simulink model "ThdRwRtStCalib"  (R2024b)
settings: Solver=FixedStepDiscrete  StartTime=0.0  StopTime=10.0  FixedStep=0.01  RelTol=1e-3
model workspace (MAT data in the model file):
  KeSMSwAcsMd7ThdRwRtStBkReclnUpwdDnwdPosMax_Val = Simulink.Parameter
  KeSMSwAcsMd7ThdRwRtStBkReclnUpwdDnwdPosMax_Val.Value = 0
  KeSMSwAcsMd7ThdRwRtStBkReclnUpwdDnwdPosMax_Val.Complexity = 'real'
  KeSMSwAcsMd7ThdRwRtStBkReclnUpwdDnwdPosMax_Val.Dimensions = [1 1]
  KeSMSwAcsMd7ThdRwRtStBkReclnUpwdDnwdPosMax_Val.DataType = 'uint16'
  KeSMSwAcsMd7ThdRwRtStBkReclnUpwdDnwdPosMin_Val = Simulink.Parameter
  KeSMSwAcsMd7ThdRwRtStBkReclnUpwdDnwdPosMin_Val.Value = 0
  KeSMSwAcsMd7ThdRwRtStBkReclnUpwdDnwdPosMin_Val.Complexity = 'real'
  KeSMSwAcsMd7ThdRwRtStBkReclnUpwdDnwdPosMin_Val.Dimensions = [1 1]
  KeSMSwAcsMd7ThdRwRtStBkReclnUpwdDnwdPosMin_Val.DataType = 'uint16'
  KeSMSwAcsMd7ThdRwRtStBkReclnUpwdDnwdPos_Val = Simulink.Parameter
  KeSMSwAcsMd7ThdRwRtStBkReclnUpwdDnwdPos_Val.Value = 0
  KeSMSwAcsMd7ThdRwRtStBkReclnUpwdDnwdPos_Val.Complexity = 'real'
  KeSMSwAcsMd7ThdRwRtStBkReclnUpwdDnwdPos_Val.Dimensions = [1 1]
  KeSMSwAcsMd7ThdRwRtStBkReclnUpwdDnwdPos_Val.DataType = 'uint16'
  KeSMSwAcsMd7ThdRwRtStCshnFldUpwdDnwdPosMax_Val = Simulink.Parameter
  KeSMSwAcsMd7ThdRwRtStCshnFldUpwdDnwdPosMax_Val.Value = 0
  KeSMSwAcsMd7ThdRwRtStCshnFldUpwdDnwdPosMax_Val.Complexity = 'real'
  KeSMSwAcsMd7ThdRwRtStCshnFldUpwdDnwdPosMax_Val.Dimensions = [1 1]
  KeSMSwAcsMd7ThdRwRtStCshnFldUpwdDnwdPosMax_Val.DataType = 'uint16'
  KeSMSwAcsMd7ThdRwRtStCshnFldUpwdDnwdPosMin_Val = Simulink.Parameter
  KeSMSwAcsMd7ThdRwRtStCshnFldUpwdDnwdPosMin_Val.Value = 0
  KeSMSwAcsMd7ThdRwRtStCshnFldUpwdDnwdPosMin_Val.Complexity = 'real'
  KeSMSwAcsMd7ThdRwRtStCshnFldUpwdDnwdPosMin_Val.Dimensions = [1 1]
  KeSMSwAcsMd7ThdRwRtStCshnFldUpwdDnwdPosMin_Val.DataType = 'uint16'
  KeSMSwAcsMd7ThdRwRtStCshnFldUpwdDnwdPos_Val = Simulink.Parameter
  KeSMSwAcsMd7ThdRwRtStCshnFldUpwdDnwdPos_Val.Value = 0
  KeSMSwAcsMd7ThdRwRtStCshnFldUpwdDnwdPos_Val.Complexity = 'real'
  KeSMSwAcsMd7ThdRwRtStCshnFldUpwdDnwdPos_Val.Dimensions = [1 1]
  KeSMSwAcsMd7ThdRwRtStCshnFldUpwdDnwdPos_Val.DataType = 'uint16'
  KeSMSwAcsMd7ThdRwRtStFrwdBkwdPosMax_Val = Simulink.Parameter
  KeSMSwAcsMd7ThdRwRtStFrwdBkwdPosMax_Val.Value = 0
  KeSMSwAcsMd7ThdRwRtStFrwdBkwdPosMax_Val.Complexity = 'real'
  KeSMSwAcsMd7ThdRwRtStFrwdBkwdPosMax_Val.Dimensions = [1 1]
  KeSMSwAcsMd7ThdRwRtStFrwdBkwdPosMax_Val.DataType = 'uint16'
  KeSMSwAcsMd7ThdRwRtStFrwdBkwdPosMin_Val = Simulink.Parameter
  KeSMSwAcsMd7ThdRwRtStFrwdBkwdPosMin_Val.Value = 0
  KeSMSwAcsMd7ThdRwRtStFrwdBkwdPosMin_Val.Complexity = 'real'
  KeSMSwAcsMd7ThdRwRtStFrwdBkwdPosMin_Val.Dimensions = [1 1]
  KeSMSwAcsMd7ThdRwRtStFrwdBkwdPosMin_Val.DataType = 'uint16'
  KeSMSwAcsMd7ThdRwRtStFrwdBkwdPos_Val = Simulink.Parameter
  KeSMSwAcsMd7ThdRwRtStFrwdBkwdPos_Val.Value = 0
  KeSMSwAcsMd7ThdRwRtStFrwdBkwdPos_Val.Complexity = 'real'
  KeSMSwAcsMd7ThdRwRtStFrwdBkwdPos_Val.Dimensions = [1 1]
  KeSMSwAcsMd7ThdRwRtStFrwdBkwdPos_Val.DataType = 'uint16'
undefined symbols (not defined in the file or in its folder): KeSMSw6sAcsEntryThdRwRtStBkReclnUpwdDnwdPos_Val, KeSMSw6sAcsEntryThdRwRtStBkReclnUpwdDnwdPosMax_Val, KeSMSw6sAcsEntryThdRwRtStBkReclnUpwdDnwdPosMin_Val, KeSMSw6sAcsEntryThdRwRtStCshnFldUpwdDnwdPos_Val, KeSMSw6sAcsEntryThdRwRtStCshnFldUpwdDnwdPosMax_Val, KeSMSw6sAcsEntryThdRwRtStCshnFldUpwdDnwdPosMin_Val, KeSMSw6sAcsEntryThdRwRtStFrwdBkwdPos_Val, KeSMSw6sAcsEntryThdRwRtStFrwdBkwdPosMax_Val, KeSMSw6sAcsEntryThdRwRtStFrwdBkwdPosMin_Val, KeSMSw6SAcsMd56ThdRwRtStBkReclnUpwdDnwdPos_Val, KeSMSw6SAcsMd56ThdRwRtStBkReclnUpwdDnwdPosMax_Val, KeSMSw6SAcsMd56ThdRwRtStBkReclnUpwdDnwdPosMin_Val, KeSMSw6SAcsMd56ThdRwRtStFrwdBkwdPos_Val, KeSMSw6SAcsMd56ThdRwRtStFrwdBkwdPosMax_Val, KeSMSw6SAcsMd56ThdRwRtStFrwdBkwdPosMin_Val, KeSMSw6SAcsMd57ThdRwRtStBkReclnUpwdDnwdPos_Val, KeSMSw6SAcsMd57ThdRwRtStBkReclnUpwdDnwdPosMax_Val, KeSMSw6SAcsMd57ThdRwRtStBkReclnUpwdDnwdPosMin_Val, KeSMSw6SAcsMd57ThdRwRtStFrwdBkwdPos_Val, KeSMSw6SAcsMd57ThdRwRtStFrwdBkwdPosMax_Val, KeSMSw6SAcsMd57ThdRwRtStFrwdBkwdPosMin_Val, KeSMSw6sFamilyMdThdRwRtStFrwdBkwdPos_Val, KeSMSw6sFamilyMdThdRwRtStFrwdBkwdPosMax_Val, KeSMSw6sFamilyMdThdRwRtStFrwdBkwdPosMin_Val, KeSMSw6sFamilyRMdThdRwRtStFrwdBkwdPos_Val, KeSMSw6sFamilyRMdThdRwRtStFrwdBkwdPosMax_Val, KeSMSw6sFamilyRMdThdRwRtStFrwdBkwdPosMin_Val, KeSMSw6sLugThdRwRtStBkReclnUpwdDnwdPos_Val, KeSMSw6sLugThdRwRtStBkReclnUpwdDnwdPosMax_Val, KeSMSw6sLugThdRwRtStBkReclnUpwdDnwdPosMin_Val, KeSMSw6sLugThdRwRtStCshnFldUpwdDnwdPos_Val, KeSMSw6sLugThdRwRtStCshnFldUpwdDnwdPosMax_Val, KeSMSw6sLugThdRwRtStCshnFldUpwdDnwdPosMin_Val, KeSMSw6sLugThdRwRtStFrwdBkwdPos_Val, KeSMSw6sLugThdRwRtStFrwdBkwdPosMax_Val, KeSMSw6sLugThdRwRtStFrwdBkwdPosMin_Val, KeSMSw6sVIPThdRwRtStBkReclnUpwdDnwdPos_Val, KeSMSw6sVIPThdRwRtStBkReclnUpwdDnwdPosMax_Val, KeSMSw6sVIPThdRwRtStBkReclnUpwdDnwdPosMin_Val, KeSMSw6sVIPThdRwRtStFrwdBkwdPos_Val, KeSMSw6sVIPThdRwRtStFrwdBkwdPosMax_Val, KeSMSw6sVIPThdRwRtStFrwdBkwdPosMin_Val, KeSMSwAcsEntryThdRwRtStBkReclnUpwdDnwdPos_Val, KeSMSwAcsEntryThdRwRtStBkReclnUpwdDnwdPosMax_Val, KeSMSwAcsEntryThdRwRtStBkReclnUpwdDnwdPosMin_Val, KeSMSwAcsEntryThdRwRtStCshnFldUpwdDnwdPos_Val, KeSMSwAcsEntryThdRwRtStCshnFldUpwdDnwdPosMax_Val, KeSMSwAcsEntryThdRwRtStCshnFldUpwdDnwdPosMin_Val, KeSMSwAcsEntryThdRwRtStFrwdBkwdPos_Val, KeSMSwAcsEntryThdRwRtStFrwdBkwdPosMax_Val, KeSMSwAcsEntryThdRwRtStFrwdBkwdPosMin_Val, KeSMSwAcsMd53ThdRwRtBkReclnUpwdDnwdPos_Val, KeSMSwAcsMd53ThdRwRtBkReclnUpwdDnwdPosMax_Val, KeSMSwAcsMd53ThdRwRtBkReclnUpwdDnwdPosMin_Val, KeSMSwAcsMd53ThdRwRtFldUpwdDnwdPos_Val, KeSMSwAcsMd53ThdRwRtFldUpwdDnwdPosMax_Val, KeSMSwAcsMd53ThdRwRtFldUpwdDnwdPosMin_Val, KeSMSwAcsMd56ThdRwRtStBkReclnUpwdDnwdPos_Val, KeSMSwAcsMd56ThdRwRtStBkReclnUpwdDnwdPosMax_Val, KeSMSwAcsMd56ThdRwRtStBkReclnUpwdDnwdPosMin_Val ... (+33)
libraries: TrgtPosSelcLib x18
(part 1 of 3)
settings Model: ParameterArgumentNames=KeSMSwAcsMd7ThdRwRtStBkReclnUpwdDnwdPosMax_Val,KeSMSwAcsMd7ThdRwRtStBkReclnUpwdDnwdPosMin_Val,KeSMSwAcsMd7ThdRwRtStBkReclnUpwdDnwdPos_Val,KeSMSwAcsMd7ThdRwRtStCshnFldUpwdDnwdPosMax_Val,KeSMSwAcsMd7ThdRwRtStCshnFldUpwdDnwdPosMin_Val,KeSMSwAcsMd7ThdRwRtStCshnFldUpwdDnwdPos_Val,KeSMSwAcsMd7ThdRwRtStFrwdBkwdPosMax_Val,KeSMSwAcsMd7ThdRwRtStFrwdBkwdPosMin_Val,KeSMSwAcsMd7ThdRwRtStFrwdBkwdPos_Val  Creator=sn2xws  LastModifiedBy=sn55gm
settings Model: ModifiedHistory=|
  | 2024.10.10 V3.5.0 增加Md57 58 增加6sBitMask
  | 2025.3.5 V3.9.0 Bug 998429 LUG模式偶发不会往前移动三排，但是报成功
settings SolverCC: AlgebraicLoopSolver=TrustRegion
settings DataIOCC: SaveFormat=StructureWithTime  ReturnWorkspaceOutputs=off
settings OptimizationCC: DefaultParameterBehavior=Inlined  EnhancedBackFolding=on  PassReuseOutputArgsAs=Individual arguments  ZeroExternalMemoryAtStartup=off  ZeroInternalMemoryAtStartup=off  OptimizeBlockOrder=speed  DifferentSizesBufferReuse=on  OptimizationCustomize=off  EfficientTunableParamExpr=on
settings DebuggingCC: ParameterTunabilityLossMsg=error  UnconnectedInputMsg=warning  UnconnectedOutputMsg=warning  UnconnectedLineMsg=warning  ArithmeticOperatorsInVariantConditions=warning
settings ModelReferenceCC: EnableRefExpFcnMdlSchedulingChecks=on
settings SFSimCC: MATLABDynamicMemAlloc=off  CustomCodeUndefinedFunction=UseInterfaceOnly
settings RTWCC: Description=AUTOSAR  SystemTargetFile=autosar.tlc  GenCodeOnly=on  TemplateMakefile=ert_default_tmf  GenerateReport=on  IncludeHyperlinkInReport=on  LaunchReport=on  DataTypeReplacement=CDataTypesFixedWidth  GenerateTraceInfo=on  GenerateTraceReport=on  GenerateTraceReportSl=on  GenerateTraceReportSf=on  GenerateTraceReportEml=on  GPUComputeCapability=3.5
settings CodeAppCC: ForceParamTrailComments=on  IgnoreCustomStorageClasses=off  OperatorAnnotations=on  SimulinkDataObjDesc=on  SFDataObjDesc=on  InsertBlockDesc=on
settings STFCustomTargetCC: TargetLangStandard=C99 (ISO)  MultiwordLength=256  ParMdlRefBuildCompliant=on  CompOptLevelCompliant=on  IncludeMdlTerminateFcn=off  CombineOutputUpdateFcns=on  SuppressErrorStatus=on  ERTCustomFileBanners=on  SupportNonFinite=off  SupportComplex=off  SupportContinuousTime=off  SupportNonInlinedSFcns=off  RemoveResetFunc=on  MATLABClassNameForMDSCustomization=Simulink.SoftwareTarget.ERTCustomization  AutosarCompliant=on  UseToolchainInfoCompliant=on  LookupTableObjectStructAxisOrder=2,1,3,4,...  LUTObjectStructOrderEvenSpacing=Size,Table,Breakpoints  SystemTargetFile=autosar.tlc
settings ERTTargetCC: TargetLangStandard=C99 (ISO)  ConcurrentExecutionCompliant=off  IncludeMdlTerminateFcn=off  SuppressErrorStatus=on  SupportNonFinite=off  SupportComplex=off  ModelStepFunctionPrototypeControlCompliant=off  CPPClassGenCompliant=off  AutosarCompliant=on  LookupTableObjectStructAxisOrder=2,1,3,4,...  LUTObjectStructOrderEvenSpacing=Size,Table,Breakpoints  ERTCustomFileTemplate=example_file_process.tlc  ERTFilePackagingFormat=Compact  BooleanTrueId=TRUE  BooleanFalseId=FALSE  DynamicArrayContainerType=coder::array

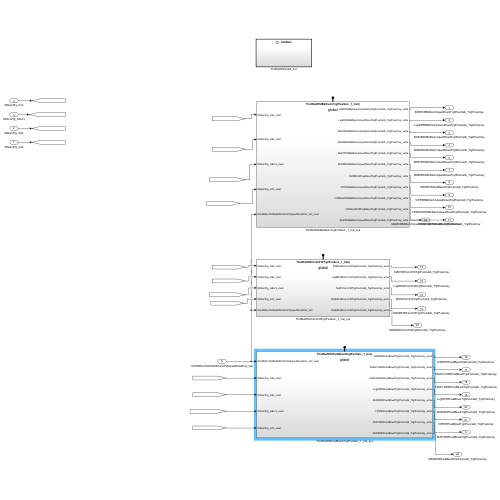
[thumbnail: Simulink's stored preview of the top-level diagram]
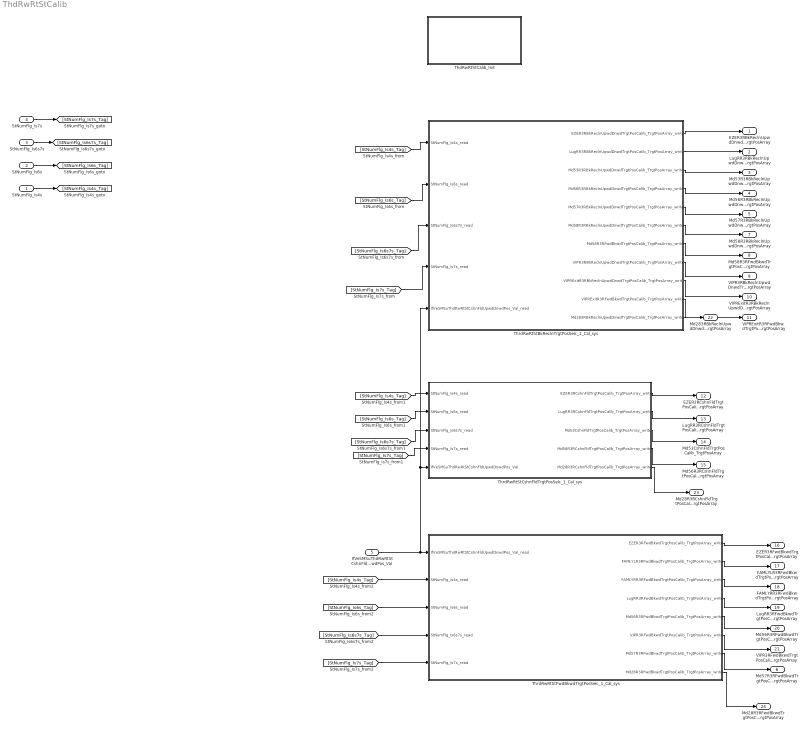
== system ThdRwRtStCalib ==
  StNumFlg_Is4s : Inport  OutDataTypeStr=boolean  PortDimensions=1
  StNumFlg_Is6s : Inport  Port=2  OutDataTypeStr=boolean  PortDimensions=1
  StNumFlg_Is6s7s : Inport  Port=3  OutDataTypeStr=boolean  PortDimensions=1
  StNumFlg_Is7s : Inport  Port=4  OutDataTypeStr=boolean  PortDimensions=1
  IfVeSMSuThdRwRtStCshnFldUpwdDnwdPos_Val : Inport  Port=5  OutDataTypeStr=uint16  PortDimensions=1
  ThdRwRtStCalib_Init : Subsystem
  ThrdRwRtStBkReclnTrgtPosSelc_1_Cal_sys : Subsystem
  ThrdRwRtStCshnFldTrgtPosSelc_1_Cal_sys : Subsystem
  ThrdRwRtStFwdBkwdTrgtPosSelc_1_Cal_sys : Subsystem
  EZER3RBkReclnUpwdDnwdTrgtPosCalib_TrgtPosArray : Outport  Description=|  OutDataTypeStr=uint16  PortDimensions=3  VectorParamsAs1DForOutWhenUnconnected=off
      | 0:Pos
      | 1:Max
      | 2:Min
  LugRR3RBkReclnUpwdDnwdTrgtPosCalib_TrgtPosArray : Outport  Description=|  Port=2  OutDataTypeStr=uint16  PortDimensions=3  VectorParamsAs1DForOutWhenUnconnected=off
      | 0:Pos
      | 1:Max
      | 2:Min
  Md53R3RBkReclnUpwdDnwdTrgtPosCalib_TrgtPosArray : Outport  Description=|  Port=3  OutDataTypeStr=uint16  PortDimensions=3  VectorParamsAs1DForOutWhenUnconnected=off
      | 0:Pos
      | 1:Max
      | 2:Min
  Md56R3RBkReclnUpwdDnwdTrgtPosCalib_TrgtPosArray : Outport  Description=|  Port=4  OutDataTypeStr=uint16  PortDimensions=3  VectorParamsAs1DForOutWhenUnconnected=off
      | 0:Pos
      | 1:Max
      | 2:Min
  Md57R3RBkReclnUpwdDnwdTrgtPosCalib_TrgtPosArray : Outport  Description=|  Port=5  OutDataTypeStr=uint16  PortDimensions=3  VectorParamsAs1DForOutWhenUnconnected=off
      | 0:Pos
      | 1:Max
      | 2:Min
  Md57R3RFwdBkwdTrgtPosCalib_TrgtPosArray : Outport  Description=|  Port=6  OutDataTypeStr=uint16  PortDimensions=3  VectorParamsAs1DForOutWhenUnconnected=off
      | 0:Pos
      | 1:Max
      | 2:Min
  Md58R3RBkReclnUpwdDnwdTrgtPosCalib_TrgtPosArray : Outport  Description=|  Port=7  OutDataTypeStr=uint16  PortDimensions=3  VectorParamsAs1DForOutWhenUnconnected=off
      | 0:Pos
      | 1:Max
      | 2:Min
  Md58R3RFwdBkwdTrgtPosCalib_TrgtPosArray : Outport  Description=|  Port=8  OutDataTypeStr=uint16  PortDimensions=3  VectorParamsAs1DForOutWhenUnconnected=off
      | 0:Pos
      | 1:Max
      | 2:Min
  VIPR3RBkReclnUpwdDnwdTrgtPosCalib_TrgtPosArray : Outport  Description=|  Port=9  OutDataTypeStr=uint16  PortDimensions=3  VectorParamsAs1DForOutWhenUnconnected=off
      | 0:Pos
      | 1:Max
      | 2:Min
  VIPRExitR3RBkReclnUpwdDnwdTrgtPosCalib_TrgtPosArray : Outport  Description=|  Port=10  OutDataTypeStr=uint16  PortDimensions=3  VectorParamsAs1DForOutWhenUnconnected=off
      | 0:Pos
      | 1:Max
      | 2:Min
  VIPRExitR3RFwdBkwdTrgtPosCalib_TrgtPosArray : Outport  Description=|  Port=11  OutDataTypeStr=uint16  PortDimensions=3  VectorParamsAs1DForOutWhenUnconnected=off
      | 0:Pos
      | 1:Max
      | 2:Min
  EZER3RCshnFldTrgtPosCalib_TrgtPosArray : Outport  Description=|  Port=12  OutDataTypeStr=uint16  PortDimensions=3  VectorParamsAs1DForOutWhenUnconnected=off
      | 0:Pos
      | 1:Max
      | 2:Min
  LugRR3RCshnFldTrgtPosCalib_TrgtPosArray : Outport  Description=|  Port=13  OutDataTypeStr=uint16  PortDimensions=3  VectorParamsAs1DForOutWhenUnconnected=off
      | 0:Pos
      | 1:Max
      | 2:Min
  Md53CshnFldTrgtPosCalib_TrgtPosArray : Outport  Description=|  Port=14  OutDataTypeStr=uint16  PortDimensions=3  VectorParamsAs1DForOutWhenUnconnected=off
      | 0:Pos
      | 1:Max
      | 2:Min
  Md56R3RCshnFldTrgtPosCalib_TrgtPosArray : Outport  Description=|  Port=15  OutDataTypeStr=uint16  PortDimensions=3  VectorParamsAs1DForOutWhenUnconnected=off
      | 0:Pos
      | 1:Max
      | 2:Min
  EZER3RFwdBkwdTrgtPosCalib_TrgtPosArray : Outport  Description=|  Port=16  OutDataTypeStr=uint16  PortDimensions=3  VectorParamsAs1DForOutWhenUnconnected=off
      | 0:Pos
      | 1:Max
      | 2:Min
  FAMLYLR3RFwdBkwdTrgtPosCalib_TrgtPosArray : Outport  Description=|  Port=17  OutDataTypeStr=uint16  PortDimensions=3  VectorParamsAs1DForOutWhenUnconnected=off
      | 0:Pos
      | 1:Max
      | 2:Min
  FAMLYRR3RFwdBkwdTrgtPosCalib_TrgtPosArray : Outport  Description=|  Port=18  OutDataTypeStr=uint16  PortDimensions=3  VectorParamsAs1DForOutWhenUnconnected=off
      | 0:Pos
      | 1:Max
      | 2:Min
  LugRR3RFwdBkwdTrgtPosCalib_TrgtPosArray : Outport  Description=|  Port=19  OutDataTypeStr=uint16  PortDimensions=3  VectorParamsAs1DForOutWhenUnconnected=off
      | 0:Pos
      | 1:Max
      | 2:Min
  Md56R3RFwdBkwdTrgtPosCalib_TrgtPosArray : Outport  Description=|  Port=20  OutDataTypeStr=uint16  PortDimensions=3  VectorParamsAs1DForOutWhenUnconnected=off
      | 0:Pos
      | 1:Max
      | 2:Min
  VIPR3RFwdBkwdTrgtPosCalib_TrgtPosArray : Outport  Description=|  Port=21  OutDataTypeStr=uint16  PortDimensions=3  VectorParamsAs1DForOutWhenUnconnected=off
      | 0:Pos
      | 1:Max
      | 2:Min
  Md283RBkReclnUpwdDnwdTrgtPosCalib_TrgtPosArray : Outport  Description=|  Port=22  OutDataTypeStr=uint16  PortDimensions=3  VectorParamsAs1DForOutWhenUnconnected=off
      | 0:Pos
      | 1:Max
      | 2:Min
  Md28R3RCshnFldTrgtPosCalib_TrgtPosArray : Outport  Description=|  Port=23  OutDataTypeStr=uint16  PortDimensions=3  VectorParamsAs1DForOutWhenUnconnected=off
      | 0:Pos
      | 1:Max
      | 2:Min
  Md28R3RFwdBkwdTrgtPosCalib_TrgtPosArray : Outport  Description=|  Port=24  OutDataTypeStr=uint16  PortDimensions=3  VectorParamsAs1DForOutWhenUnconnected=off
      | 0:Pos
      | 1:Max
      | 2:Min
  wires:
  ThrdRwRtStBkReclnTrgtPosSelc_1_Cal_sys/1(EZER3RBkReclnUpwdDnwdTrgtPosCalib_TrgtPosArray_write) -> EZER3RBkReclnUpwdDnwdTrgtPosCalib_TrgtPosArray/1
  ThrdRwRtStBkReclnTrgtPosSelc_1_Cal_sys/2(LugRR3RBkReclnUpwdDnwdTrgtPosCalib_TrgtPosArray_write) -> LugRR3RBkReclnUpwdDnwdTrgtPosCalib_TrgtPosArray/1
  ThrdRwRtStBkReclnTrgtPosSelc_1_Cal_sys/3(Md53R3RBkReclnUpwdDnwdTrgtPosCalib_TrgtPosArray_write) -> Md53R3RBkReclnUpwdDnwdTrgtPosCalib_TrgtPosArray/1
  ThrdRwRtStBkReclnTrgtPosSelc_1_Cal_sys/4(Md56R3RBkReclnUpwdDnwdTrgtPosCalib_TrgtPosArray_write) -> Md56R3RBkReclnUpwdDnwdTrgtPosCalib_TrgtPosArray/1
  ThrdRwRtStBkReclnTrgtPosSelc_1_Cal_sys/5(Md57R3RBkReclnUpwdDnwdTrgtPosCalib_TrgtPosArray_write) -> Md57R3RBkReclnUpwdDnwdTrgtPosCalib_TrgtPosArray/1
  ThrdRwRtStBkReclnTrgtPosSelc_1_Cal_sys/6(Md58R3RBkReclnUpwdDnwdTrgtPosCalib_TrgtPosArray_write) -> Md58R3RBkReclnUpwdDnwdTrgtPosCalib_TrgtPosArray/1
  ThrdRwRtStBkReclnTrgtPosSelc_1_Cal_sys/7(Md58R3RFwdBkwdTrgtPosCalib_TrgtPosArray_write) -> Md58R3RFwdBkwdTrgtPosCalib_TrgtPosArray/1
  ThrdRwRtStBkReclnTrgtPosSelc_1_Cal_sys/8(VIPR3RBkReclnUpwdDnwdTrgtPosCalib_TrgtPosArray_write) -> VIPR3RBkReclnUpwdDnwdTrgtPosCalib_TrgtPosArray/1
  ThrdRwRtStBkReclnTrgtPosSelc_1_Cal_sys/9(VIPRExitR3RBkReclnUpwdDnwdTrgtPosCalib_TrgtPosArray_write) -> VIPRExitR3RBkReclnUpwdDnwdTrgtPosCalib_TrgtPosArray/1
  ThrdRwRtStBkReclnTrgtPosSelc_1_Cal_sys/10(VIPRExitR3RFwdBkwdTrgtPosCalib_TrgtPosArray_write) -> VIPRExitR3RFwdBkwdTrgtPosCalib_TrgtPosArray/1
  ThrdRwRtStCshnFldTrgtPosSelc_1_Cal_sys/1(EZER3RCshnFldTrgtPosCalib_TrgtPosArray_write) -> EZER3RCshnFldTrgtPosCalib_TrgtPosArray/1
  ThrdRwRtStCshnFldTrgtPosSelc_1_Cal_sys/2(LugRR3RCshnFldTrgtPosCalib_TrgtPosArray_write) -> LugRR3RCshnFldTrgtPosCalib_TrgtPosArray/1
  ThrdRwRtStCshnFldTrgtPosSelc_1_Cal_sys/3(Md53CshnFldTrgtPosCalib_TrgtPosArray_write) -> Md53CshnFldTrgtPosCalib_TrgtPosArray/1
  ThrdRwRtStCshnFldTrgtPosSelc_1_Cal_sys/4(Md56R3RCshnFldTrgtPosCalib_TrgtPosArray_write) -> Md56R3RCshnFldTrgtPosCalib_TrgtPosArray/1
  IfVeSMSuThdRwRtStCshnFldUpwdDnwdPos_Val/1 -> ThrdRwRtStCshnFldTrgtPosSelc_1_Cal_sys/5(IfVeSMSuThdRwRtStCshnFldUpwdDnwdPos_Val), ThrdRwRtStBkReclnTrgtPosSelc_1_Cal_sys/5(IfVeSMSuThdRwRtStCshnFldUpwdDnwdPos_Val_read), ThrdRwRtStFwdBkwdTrgtPosSelc_1_Cal_sys/1(IfVeSMSuThdRwRtStCshnFldUpwdDnwdPos_Val_read)
  ThrdRwRtStFwdBkwdTrgtPosSelc_1_Cal_sys/1(EZER3RFwdBkwdTrgtPosCalib_TrgtPosArray_write) -> EZER3RFwdBkwdTrgtPosCalib_TrgtPosArray/1
  ThrdRwRtStFwdBkwdTrgtPosSelc_1_Cal_sys/2(FAMLYLR3RFwdBkwdTrgtPosCalib_TrgtPosArray_write) -> FAMLYLR3RFwdBkwdTrgtPosCalib_TrgtPosArray/1
  ThrdRwRtStFwdBkwdTrgtPosSelc_1_Cal_sys/3(FAMLYRR3RFwdBkwdTrgtPosCalib_TrgtPosArray_write) -> FAMLYRR3RFwdBkwdTrgtPosCalib_TrgtPosArray/1
  ThrdRwRtStFwdBkwdTrgtPosSelc_1_Cal_sys/4(LugRR3RFwdBkwdTrgtPosCalib_TrgtPosArray_write) -> LugRR3RFwdBkwdTrgtPosCalib_TrgtPosArray/1
  ThrdRwRtStFwdBkwdTrgtPosSelc_1_Cal_sys/5(Md56R3RFwdBkwdTrgtPosCalib_TrgtPosArray_write) -> Md56R3RFwdBkwdTrgtPosCalib_TrgtPosArray/1
  ThrdRwRtStFwdBkwdTrgtPosSelc_1_Cal_sys/6(VIPR3RFwdBkwdTrgtPosCalib_TrgtPosArray_write) -> VIPR3RFwdBkwdTrgtPosCalib_TrgtPosArray/1
  StNumFlg_Is7s/1 -> [StNumFlg_Is7s_Tag]
  [StNumFlg_Is7s_Tag] -> ThrdRwRtStBkReclnTrgtPosSelc_1_Cal_sys/4(StNumFlg_Is7s_read)
  [StNumFlg_Is7s_Tag] -> ThrdRwRtStCshnFldTrgtPosSelc_1_Cal_sys/4(StNumFlg_Is7s_read)
  [StNumFlg_Is7s_Tag] -> ThrdRwRtStFwdBkwdTrgtPosSelc_1_Cal_sys/5(StNumFlg_Is7s_read)
  StNumFlg_Is6s7s/1 -> [StNumFlg_Is6s7s_Tag]
  [StNumFlg_Is6s7s_Tag] -> ThrdRwRtStBkReclnTrgtPosSelc_1_Cal_sys/3(StNumFlg_Is6s7s_read)
  [StNumFlg_Is6s7s_Tag] -> ThrdRwRtStCshnFldTrgtPosSelc_1_Cal_sys/3(StNumFlg_Is6s7s_read)
  [StNumFlg_Is6s7s_Tag] -> ThrdRwRtStFwdBkwdTrgtPosSelc_1_Cal_sys/4(StNumFlg_Is6s7s_read)
  StNumFlg_Is6s/1 -> [StNumFlg_Is6s_Tag]
  [StNumFlg_Is6s_Tag] -> ThrdRwRtStBkReclnTrgtPosSelc_1_Cal_sys/2(StNumFlg_Is6s_read)
  [StNumFlg_Is6s_Tag] -> ThrdRwRtStCshnFldTrgtPosSelc_1_Cal_sys/2(StNumFlg_Is6s_read)
  [StNumFlg_Is6s_Tag] -> ThrdRwRtStFwdBkwdTrgtPosSelc_1_Cal_sys/3(StNumFlg_Is6s_read)
  StNumFlg_Is4s/1 -> [StNumFlg_Is4s_Tag]
  [StNumFlg_Is4s_Tag] -> ThrdRwRtStBkReclnTrgtPosSelc_1_Cal_sys/1(StNumFlg_Is4s_read)
  [StNumFlg_Is4s_Tag] -> ThrdRwRtStCshnFldTrgtPosSelc_1_Cal_sys/1(StNumFlg_Is4s_read)
  [StNumFlg_Is4s_Tag] -> ThrdRwRtStFwdBkwdTrgtPosSelc_1_Cal_sys/2(StNumFlg_Is4s_read)
  ThrdRwRtStFwdBkwdTrgtPosSelc_1_Cal_sys/7(Md57R3RFwdBkwdTrgtPosCalib_TrgtPosArray_write) -> Md57R3RFwdBkwdTrgtPosCalib_TrgtPosArray/1
  ThrdRwRtStBkReclnTrgtPosSelc_1_Cal_sys/11(Md283RBkReclnUpwdDnwdTrgtPosCalib_TrgtPosArray_write) -> Md283RBkReclnUpwdDnwdTrgtPosCalib_TrgtPosArray/1
  ThrdRwRtStCshnFldTrgtPosSelc_1_Cal_sys/5(Md28R3RCshnFldTrgtPosCalib_TrgtPosArray_write) -> Md28R3RCshnFldTrgtPosCalib_TrgtPosArray/1
  ThrdRwRtStFwdBkwdTrgtPosSelc_1_Cal_sys/8(Md28R3RFwdBkwdTrgtPosCalib_TrgtPosArray_write) -> Md28R3RFwdBkwdTrgtPosCalib_TrgtPosArray/1

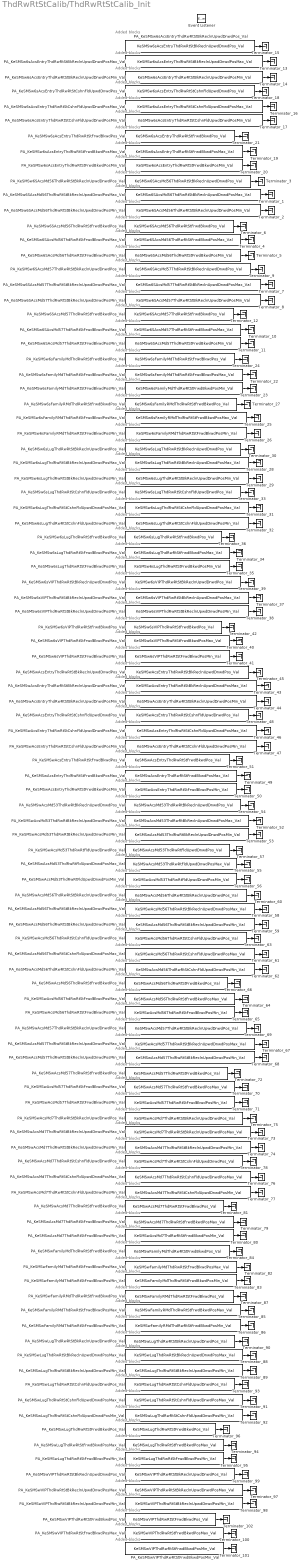
== system ThdRwRtStCalib/ThdRwRtStCalib_Init ==
  note: Added blocks
  note: Added blocks
  note: Added blocks
  note: Added blocks
  note: Added blocks
  note: Added blocks
  note: Added blocks
  note: Added blocks
  note: Added blocks
  note: Added blocks
  note: Added blocks
  note: Added blocks
  note: Added blocks
  note: Added blocks
  note: Added blocks
  note: Added blocks
  note: Added blocks
  note: Added blocks
  note: Added blocks
  note: Added blocks
  note: Added blocks
  note: Added blocks
  note: Added blocks
  note: Added blocks
  note: Added blocks
  note: Added blocks
  note: Added blocks
  note: Added blocks
  note: Added blocks
  note: Added blocks
  note: Added blocks
  note: Added blocks
  note: Added blocks
  note: Added blocks
  note: Added blocks
  note: Added blocks
  note: Added blocks
  note: Added blocks
  note: Added blocks
  note: Added blocks
  note: Added blocks
  note: Added blocks
  note: Added blocks
  note: Added blocks
  note: Added blocks
  note: Added blocks
  note: Added blocks
  note: Added blocks
  note: Added blocks
  note: Added blocks
  note: Added blocks
  note: Added blocks
  note: Added blocks
  note: Added blocks
  note: Added blocks
  note: Added blocks
  note: Added blocks
  note: Added blocks
  note: Added blocks
  note: Added blocks
  note: Added blocks
  note: Added blocks
  note: Added blocks
  note: Added blocks
  note: Added blocks
  note: Added blocks
  note: Added blocks
  note: Added blocks
  note: Added blocks
  note: Added blocks
  note: Added blocks
  note: Added blocks
  note: Added blocks
  note: Added blocks
  note: Added blocks
  note: Added blocks
  note: Added blocks
  note: Added blocks
  note: Added blocks
  note: Added blocks
  note: Added blocks
  note: Added blocks
  note: Added blocks
  note: Added blocks
  note: Added blocks
  note: Added blocks
  note: Added blocks
  note: Added blocks
  note: Added blocks
  note: Added blocks
  note: Added blocks
  note: Added blocks
  note: Added blocks
  note: Added blocks
  note: Added blocks
  note: Added blocks
  note: Added blocks
  note: Added blocks
  note: Added blocks
  note: Added blocks
  note: Added blocks
  note: Added blocks
  Event Listener : EventListener  EventName=reset
  PA_KeSMSw6SAcsMd56ThdRwRtStBkReclnUpwdDnwdPosMax_Val : Constant  Value=KeSMSw6SAcsMd56ThdRwRtStBkReclnUpwdDnwdPosMax_Val
  PA_KeSMSw6SAcsMd56ThdRwRtStBkReclnUpwdDnwdPosMin_Val : Constant  Value=KeSMSw6SAcsMd56ThdRwRtStBkReclnUpwdDnwdPosMin_Val
  PA_KeSMSw6SAcsMd56ThdRwRtStBkReclnUpwdDnwdPos_Val : Constant  Value=KeSMSw6SAcsMd56ThdRwRtStBkReclnUpwdDnwdPos_Val
  PA_KeSMSw6SAcsMd56ThdRwRtStFrwdBkwdPosMax_Val : Constant  Value=KeSMSw6SAcsMd56ThdRwRtStFrwdBkwdPosMax_Val
  PA_KeSMSw6SAcsMd56ThdRwRtStFrwdBkwdPosMin_Val : Constant  Value=KeSMSw6SAcsMd56ThdRwRtStFrwdBkwdPosMin_Val
  PA_KeSMSw6SAcsMd56ThdRwRtStFrwdBkwdPos_Val : Constant  Value=KeSMSw6SAcsMd56ThdRwRtStFrwdBkwdPos_Val
  PA_KeSMSw6SAcsMd57ThdRwRtStBkReclnUpwdDnwdPosMax_Val : Constant  Value=KeSMSw6SAcsMd57ThdRwRtStBkReclnUpwdDnwdPosMax_Val
  PA_KeSMSw6SAcsMd57ThdRwRtStBkReclnUpwdDnwdPosMin_Val : Constant  Value=KeSMSw6SAcsMd57ThdRwRtStBkReclnUpwdDnwdPosMin_Val
  PA_KeSMSw6SAcsMd57ThdRwRtStBkReclnUpwdDnwdPos_Val : Constant  Value=KeSMSw6SAcsMd57ThdRwRtStBkReclnUpwdDnwdPos_Val
  PA_KeSMSw6SAcsMd57ThdRwRtStFrwdBkwdPosMax_Val : Constant  Value=KeSMSw6SAcsMd57ThdRwRtStFrwdBkwdPosMax_Val
  PA_KeSMSw6SAcsMd57ThdRwRtStFrwdBkwdPosMin_Val : Constant  Value=KeSMSw6SAcsMd57ThdRwRtStFrwdBkwdPosMin_Val
  PA_KeSMSw6SAcsMd57ThdRwRtStFrwdBkwdPos_Val : Constant  Value=KeSMSw6SAcsMd57ThdRwRtStFrwdBkwdPos_Val
  PA_KeSMSw6sAcsEntryThdRwRtStBkReclnUpwdDnwdPosMax_Val : Constant  Value=KeSMSw6sAcsEntryThdRwRtStBkReclnUpwdDnwdPosMax_Val
  PA_KeSMSw6sAcsEntryThdRwRtStBkReclnUpwdDnwdPosMin_Val : Constant  Value=KeSMSw6sAcsEntryThdRwRtStBkReclnUpwdDnwdPosMin_Val
  PA_KeSMSw6sAcsEntryThdRwRtStBkReclnUpwdDnwdPos_Val : Constant  Value=KeSMSw6sAcsEntryThdRwRtStBkReclnUpwdDnwdPos_Val
  PA_KeSMSw6sAcsEntryThdRwRtStCshnFldUpwdDnwdPosMax_Val : Constant  Value=KeSMSw6sAcsEntryThdRwRtStCshnFldUpwdDnwdPosMax_Val
  PA_KeSMSw6sAcsEntryThdRwRtStCshnFldUpwdDnwdPosMin_Val : Constant  Value=KeSMSw6sAcsEntryThdRwRtStCshnFldUpwdDnwdPosMin_Val
  PA_KeSMSw6sAcsEntryThdRwRtStCshnFldUpwdDnwdPos_Val : Constant  Value=KeSMSw6sAcsEntryThdRwRtStCshnFldUpwdDnwdPos_Val
  PA_KeSMSw6sAcsEntryThdRwRtStFrwdBkwdPosMax_Val : Constant  Value=KeSMSw6sAcsEntryThdRwRtStFrwdBkwdPosMax_Val
  PA_KeSMSw6sAcsEntryThdRwRtStFrwdBkwdPosMin_Val : Constant  Value=KeSMSw6sAcsEntryThdRwRtStFrwdBkwdPosMin_Val
  PA_KeSMSw6sAcsEntryThdRwRtStFrwdBkwdPos_Val : Constant  Value=KeSMSw6sAcsEntryThdRwRtStFrwdBkwdPos_Val
  PA_KeSMSw6sFamilyMdThdRwRtStFrwdBkwdPosMax_Val : Constant  Value=KeSMSw6sFamilyMdThdRwRtStFrwdBkwdPosMax_Val
  PA_KeSMSw6sFamilyMdThdRwRtStFrwdBkwdPosMin_Val : Constant  Value=KeSMSw6sFamilyMdThdRwRtStFrwdBkwdPosMin_Val
  PA_KeSMSw6sFamilyMdThdRwRtStFrwdBkwdPos_Val : Constant  Value=KeSMSw6sFamilyMdThdRwRtStFrwdBkwdPos_Val
  PA_KeSMSw6sFamilyRMdThdRwRtStFrwdBkwdPosMax_Val : Constant  Value=KeSMSw6sFamilyRMdThdRwRtStFrwdBkwdPosMax_Val
  PA_KeSMSw6sFamilyRMdThdRwRtStFrwdBkwdPosMin_Val : Constant  Value=KeSMSw6sFamilyRMdThdRwRtStFrwdBkwdPosMin_Val
  PA_KeSMSw6sFamilyRMdThdRwRtStFrwdBkwdPos_Val : Constant  Value=KeSMSw6sFamilyRMdThdRwRtStFrwdBkwdPos_Val
  PA_KeSMSw6sLugThdRwRtStBkReclnUpwdDnwdPosMax_Val : Constant  Value=KeSMSw6sLugThdRwRtStBkReclnUpwdDnwdPosMax_Val
  PA_KeSMSw6sLugThdRwRtStBkReclnUpwdDnwdPosMin_Val : Constant  Value=KeSMSw6sLugThdRwRtStBkReclnUpwdDnwdPosMin_Val
  PA_KeSMSw6sLugThdRwRtStBkReclnUpwdDnwdPos_Val : Constant  Value=KeSMSw6sLugThdRwRtStBkReclnUpwdDnwdPos_Val
  PA_KeSMSw6sLugThdRwRtStCshnFldUpwdDnwdPosMax_Val : Constant  Value=KeSMSw6sLugThdRwRtStCshnFldUpwdDnwdPosMax_Val
  PA_KeSMSw6sLugThdRwRtStCshnFldUpwdDnwdPosMin_Val : Constant  Value=KeSMSw6sLugThdRwRtStCshnFldUpwdDnwdPosMin_Val
  PA_KeSMSw6sLugThdRwRtStCshnFldUpwdDnwdPos_Val : Constant  Value=KeSMSw6sLugThdRwRtStCshnFldUpwdDnwdPos_Val
  PA_KeSMSw6sLugThdRwRtStFrwdBkwdPosMax_Val : Constant  Value=KeSMSw6sLugThdRwRtStFrwdBkwdPosMax_Val
  PA_KeSMSw6sLugThdRwRtStFrwdBkwdPosMin_Val : Constant  Value=KeSMSw6sLugThdRwRtStFrwdBkwdPosMin_Val
  PA_KeSMSw6sLugThdRwRtStFrwdBkwdPos_Val : Constant  Value=KeSMSw6sLugThdRwRtStFrwdBkwdPos_Val
  PA_KeSMSw6sVIPThdRwRtStBkReclnUpwdDnwdPosMax_Val : Constant  Value=KeSMSw6sVIPThdRwRtStBkReclnUpwdDnwdPosMax_Val
  PA_KeSMSw6sVIPThdRwRtStBkReclnUpwdDnwdPosMin_Val : Constant  Value=KeSMSw6sVIPThdRwRtStBkReclnUpwdDnwdPosMin_Val
  PA_KeSMSw6sVIPThdRwRtStBkReclnUpwdDnwdPos_Val : Constant  Value=KeSMSw6sVIPThdRwRtStBkReclnUpwdDnwdPos_Val
  PA_KeSMSw6sVIPThdRwRtStFrwdBkwdPosMax_Val : Constant  Value=KeSMSw6sVIPThdRwRtStFrwdBkwdPosMax_Val
  PA_KeSMSw6sVIPThdRwRtStFrwdBkwdPosMin_Val : Constant  Value=KeSMSw6sVIPThdRwRtStFrwdBkwdPosMin_Val
  PA_KeSMSw6sVIPThdRwRtStFrwdBkwdPos_Val : Constant  Value=KeSMSw6sVIPThdRwRtStFrwdBkwdPos_Val
  PA_KeSMSwAcsEntryThdRwRtStBkReclnUpwdDnwdPosMax_Val : Constant  Value=KeSMSwAcsEntryThdRwRtStBkReclnUpwdDnwdPosMax_Val
  PA_KeSMSwAcsEntryThdRwRtStBkReclnUpwdDnwdPosMin_Val : Constant  Value=KeSMSwAcsEntryThdRwRtStBkReclnUpwdDnwdPosMin_Val
  PA_KeSMSwAcsEntryThdRwRtStBkReclnUpwdDnwdPos_Val : Constant  Value=KeSMSwAcsEntryThdRwRtStBkReclnUpwdDnwdPos_Val
  PA_KeSMSwAcsEntryThdRwRtStCshnFldUpwdDnwdPosMax_Val : Constant  Value=KeSMSwAcsEntryThdRwRtStCshnFldUpwdDnwdPosMax_Val
  PA_KeSMSwAcsEntryThdRwRtStCshnFldUpwdDnwdPosMin_Val : Constant  Value=KeSMSwAcsEntryThdRwRtStCshnFldUpwdDnwdPosMin_Val
  PA_KeSMSwAcsEntryThdRwRtStCshnFldUpwdDnwdPos_Val : Constant  Value=KeSMSwAcsEntryThdRwRtStCshnFldUpwdDnwdPos_Val
  PA_KeSMSwAcsEntryThdRwRtStFrwdBkwdPosMax_Val : Constant  Value=KeSMSwAcsEntryThdRwRtStFrwdBkwdPosMax_Val
  PA_KeSMSwAcsEntryThdRwRtStFrwdBkwdPosMin_Val : Constant  Value=KeSMSwAcsEntryThdRwRtStFrwdBkwdPosMin_Val
  PA_KeSMSwAcsEntryThdRwRtStFrwdBkwdPos_Val : Constant  Value=KeSMSwAcsEntryThdRwRtStFrwdBkwdPos_Val
  PA_KeSMSwAcsMd53ThdRwRtBkReclnUpwdDnwdPosMax_Val : Constant  Value=KeSMSwAcsMd53ThdRwRtBkReclnUpwdDnwdPosMax_Val
  PA_KeSMSwAcsMd53ThdRwRtBkReclnUpwdDnwdPosMin_Val : Constant  Value=KeSMSwAcsMd53ThdRwRtBkReclnUpwdDnwdPosMin_Val
  PA_KeSMSwAcsMd53ThdRwRtBkReclnUpwdDnwdPos_Val : Constant  Value=KeSMSwAcsMd53ThdRwRtBkReclnUpwdDnwdPos_Val
  PA_KeSMSwAcsMd53ThdRwRtFldUpwdDnwdPosMax_Val : Constant  Value=KeSMSwAcsMd53ThdRwRtFldUpwdDnwdPosMax_Val
  PA_KeSMSwAcsMd53ThdRwRtFldUpwdDnwdPosMin_Val : Constant  Value=KeSMSwAcsMd53ThdRwRtFldUpwdDnwdPosMin_Val
  PA_KeSMSwAcsMd53ThdRwRtFldUpwdDnwdPos_Val : Constant  Value=KeSMSwAcsMd53ThdRwRtFldUpwdDnwdPos_Val
  PA_KeSMSwAcsMd56ThdRwRtStBkReclnUpwdDnwdPosMax_Val : Constant  Value=KeSMSwAcsMd56ThdRwRtStBkReclnUpwdDnwdPosMax_Val
  PA_KeSMSwAcsMd56ThdRwRtStBkReclnUpwdDnwdPosMin_Val : Constant  Value=KeSMSwAcsMd56ThdRwRtStBkReclnUpwdDnwdPosMin_Val
  PA_KeSMSwAcsMd56ThdRwRtStBkReclnUpwdDnwdPos_Val : Constant  Value=KeSMSwAcsMd56ThdRwRtStBkReclnUpwdDnwdPos_Val
  PA_KeSMSwAcsMd56ThdRwRtStCshnFldUpwdDnwdPosMax_Val : Constant  Value=KeSMSwAcsMd56ThdRwRtStCshnFldUpwdDnwdPosMax_Val
  PA_KeSMSwAcsMd56ThdRwRtStCshnFldUpwdDnwdPosMin_Val : Constant  Value=KeSMSwAcsMd56ThdRwRtStCshnFldUpwdDnwdPosMin_Val
  PA_KeSMSwAcsMd56ThdRwRtStCshnFldUpwdDnwdPos_Val : Constant  Value=KeSMSwAcsMd56ThdRwRtStCshnFldUpwdDnwdPos_Val
  PA_KeSMSwAcsMd56ThdRwRtStFrwdBkwdPosMax_Val : Constant  Value=KeSMSwAcsMd56ThdRwRtStFrwdBkwdPosMax_Val
  PA_KeSMSwAcsMd56ThdRwRtStFrwdBkwdPosMin_Val : Constant  Value=KeSMSwAcsMd56ThdRwRtStFrwdBkwdPosMin_Val
  PA_KeSMSwAcsMd56ThdRwRtStFrwdBkwdPos_Val : Constant  Value=KeSMSwAcsMd56ThdRwRtStFrwdBkwdPos_Val
  PA_KeSMSwAcsMd57ThdRwRtStBkReclnUpwdDnwdPosMax_Val : Constant  Value=KeSMSwAcsMd57ThdRwRtStBkReclnUpwdDnwdPosMax_Val
  PA_KeSMSwAcsMd57ThdRwRtStBkReclnUpwdDnwdPosMin_Val : Constant  Value=KeSMSwAcsMd57ThdRwRtStBkReclnUpwdDnwdPosMin_Val
  PA_KeSMSwAcsMd57ThdRwRtStBkReclnUpwdDnwdPos_Val : Constant  Value=KeSMSwAcsMd57ThdRwRtStBkReclnUpwdDnwdPos_Val
  PA_KeSMSwAcsMd57ThdRwRtStFrwdBkwdPosMax_Val : Constant  Value=KeSMSwAcsMd57ThdRwRtStFrwdBkwdPosMax_Val
  PA_KeSMSwAcsMd57ThdRwRtStFrwdBkwdPosMin_Val : Constant  Value=KeSMSwAcsMd57ThdRwRtStFrwdBkwdPosMin_Val
  PA_KeSMSwAcsMd57ThdRwRtStFrwdBkwdPos_Val : Constant  Value=KeSMSwAcsMd57ThdRwRtStFrwdBkwdPos_Val
  PA_KeSMSwAcsMd7ThdRwRtStBkReclnUpwdDnwdPosMax_Val : Constant  Value=KeSMSwAcsMd7ThdRwRtStBkReclnUpwdDnwdPosMax_Val
  PA_KeSMSwAcsMd7ThdRwRtStBkReclnUpwdDnwdPosMin_Val : Constant  Value=KeSMSwAcsMd7ThdRwRtStBkReclnUpwdDnwdPosMin_Val
  PA_KeSMSwAcsMd7ThdRwRtStBkReclnUpwdDnwdPos_Val : Constant  Value=KeSMSwAcsMd7ThdRwRtStBkReclnUpwdDnwdPos_Val
  PA_KeSMSwAcsMd7ThdRwRtStCshnFldUpwdDnwdPosMax_Val : Constant  Value=KeSMSwAcsMd7ThdRwRtStCshnFldUpwdDnwdPosMax_Val
  PA_KeSMSwAcsMd7ThdRwRtStCshnFldUpwdDnwdPosMin_Val : Constant  Value=KeSMSwAcsMd7ThdRwRtStCshnFldUpwdDnwdPosMin_Val
  PA_KeSMSwAcsMd7ThdRwRtStCshnFldUpwdDnwdPos_Val : Constant  Value=KeSMSwAcsMd7ThdRwRtStCshnFldUpwdDnwdPos_Val
  PA_KeSMSwAcsMd7ThdRwRtStFrwdBkwdPosMax_Val : Constant  Value=KeSMSwAcsMd7ThdRwRtStFrwdBkwdPosMax_Val
  PA_KeSMSwAcsMd7ThdRwRtStFrwdBkwdPosMin_Val : Constant  Value=KeSMSwAcsMd7ThdRwRtStFrwdBkwdPosMin_Val
  PA_KeSMSwAcsMd7ThdRwRtStFrwdBkwdPos_Val : Constant  Value=KeSMSwAcsMd7ThdRwRtStFrwdBkwdPos_Val
  PA_KeSMSwFamilyMdThdRwRtStFrwdBkwdPosMax_Val : Constant  Value=KeSMSwFamilyMdThdRwRtStFrwdBkwdPosMax_Val
  PA_KeSMSwFamilyMdThdRwRtStFrwdBkwdPosMin_Val : Constant  Value=KeSMSwFamilyMdThdRwRtStFrwdBkwdPosMin_Val
  PA_KeSMSwFamilyMdThdRwRtStFrwdBkwdPos_Val : Constant  Value=KeSMSwFamilyMdThdRwRtStFrwdBkwdPos_Val
  PA_KeSMSwFamilyRMdThdRwRtStFrwdBkwdPosMax_Val : Constant  Value=KeSMSwFamilyRMdThdRwRtStFrwdBkwdPosMax_Val
  PA_KeSMSwFamilyRMdThdRwRtStFrwdBkwdPosMin_Val : Constant  Value=KeSMSwFamilyRMdThdRwRtStFrwdBkwdPosMin_Val
  PA_KeSMSwFamilyRMdThdRwRtStFrwdBkwdPos_Val : Constant  Value=KeSMSwFamilyRMdThdRwRtStFrwdBkwdPos_Val
  PA_KeSMSwLugThdRwRtStBkReclnUpwdDnwdPosMax_Val : Constant  Value=KeSMSwLugThdRwRtStBkReclnUpwdDnwdPosMax_Val
  PA_KeSMSwLugThdRwRtStBkReclnUpwdDnwdPosMin_Val : Constant  Value=KeSMSwLugThdRwRtStBkReclnUpwdDnwdPosMin_Val
  PA_KeSMSwLugThdRwRtStBkReclnUpwdDnwdPos_Val : Constant  Value=KeSMSwLugThdRwRtStBkReclnUpwdDnwdPos_Val
  PA_KeSMSwLugThdRwRtStCshnFldUpwdDnwdPosMax_Val : Constant  Value=KeSMSwLugThdRwRtStCshnFldUpwdDnwdPosMax_Val
  PA_KeSMSwLugThdRwRtStCshnFldUpwdDnwdPosMin_Val : Constant  Value=KeSMSwLugThdRwRtStCshnFldUpwdDnwdPosMin_Val
  PA_KeSMSwLugThdRwRtStCshnFldUpwdDnwdPos_Val : Constant  Value=KeSMSwLugThdRwRtStCshnFldUpwdDnwdPos_Val
  PA_KeSMSwLugThdRwRtStFrwdBkwdPosMax_Val : Constant  Value=KeSMSwLugThdRwRtStFrwdBkwdPosMax_Val
  PA_KeSMSwLugThdRwRtStFrwdBkwdPosMin_Val : Constant  Value=KeSMSwLugThdRwRtStFrwdBkwdPosMin_Val
  PA_KeSMSwLugThdRwRtStFrwdBkwdPos_Val : Constant  Value=KeSMSwLugThdRwRtStFrwdBkwdPos_Val
  PA_KeSMSwVIPThdRwRtStBkReclnUpwdDnwdPosMax_Val : Constant  Value=KeSMSwVIPThdRwRtStBkReclnUpwdDnwdPosMax_Val
  PA_KeSMSwVIPThdRwRtStBkReclnUpwdDnwdPosMin_Val : Constant  Value=KeSMSwVIPThdRwRtStBkReclnUpwdDnwdPosMin_Val
  PA_KeSMSwVIPThdRwRtStBkReclnUpwdDnwdPos_Val : Constant  Value=KeSMSwVIPThdRwRtStBkReclnUpwdDnwdPos_Val
  PA_KeSMSwVIPThdRwRtStFrwdBkwdPosMax_Val : Constant  Value=KeSMSwVIPThdRwRtStFrwdBkwdPosMax_Val
  PA_KeSMSwVIPThdRwRtStFrwdBkwdPosMin_Val : Constant  Value=KeSMSwVIPThdRwRtStFrwdBkwdPosMin_Val
  PA_KeSMSwVIPThdRwRtStFrwdBkwdPos_Val : Constant  Value=KeSMSwVIPThdRwRtStFrwdBkwdPos_Val
  Terminator_{1..102} (102 alike) : Terminator
  wires:
  PA_KeSMSw6SAcsMd56ThdRwRtStBkReclnUpwdDnwdPosMax_Val/1 -> Terminator_1/1
  PA_KeSMSw6SAcsMd56ThdRwRtStBkReclnUpwdDnwdPosMin_Val/1 -> Terminator_2/1
  PA_KeSMSw6SAcsMd56ThdRwRtStBkReclnUpwdDnwdPos_Val/1 -> Terminator_3/1
  PA_KeSMSw6SAcsMd56ThdRwRtStFrwdBkwdPosMax_Val/1 -> Terminator_4/1
  PA_KeSMSw6SAcsMd56ThdRwRtStFrwdBkwdPosMin_Val/1 -> Terminator_5/1
  PA_KeSMSw6SAcsMd56ThdRwRtStFrwdBkwdPos_Val/1 -> Terminator_6/1
  PA_KeSMSw6SAcsMd57ThdRwRtStBkReclnUpwdDnwdPosMax_Val/1 -> Terminator_7/1
  PA_KeSMSw6SAcsMd57ThdRwRtStBkReclnUpwdDnwdPosMin_Val/1 -> Terminator_8/1
  PA_KeSMSw6SAcsMd57ThdRwRtStBkReclnUpwdDnwdPos_Val/1 -> Terminator_9/1
  PA_KeSMSw6SAcsMd57ThdRwRtStFrwdBkwdPosMax_Val/1 -> Terminator_10/1
  PA_KeSMSw6SAcsMd57ThdRwRtStFrwdBkwdPosMin_Val/1 -> Terminator_11/1
  PA_KeSMSw6SAcsMd57ThdRwRtStFrwdBkwdPos_Val/1 -> Terminator_12/1
  PA_KeSMSw6sAcsEntryThdRwRtStBkReclnUpwdDnwdPosMax_Val/1 -> Terminator_13/1
  PA_KeSMSw6sAcsEntryThdRwRtStBkReclnUpwdDnwdPosMin_Val/1 -> Terminator_14/1
  PA_KeSMSw6sAcsEntryThdRwRtStBkReclnUpwdDnwdPos_Val/1 -> Terminator_15/1
  PA_KeSMSw6sAcsEntryThdRwRtStCshnFldUpwdDnwdPosMax_Val/1 -> Terminator_16/1
  PA_KeSMSw6sAcsEntryThdRwRtStCshnFldUpwdDnwdPosMin_Val/1 -> Terminator_17/1
  PA_KeSMSw6sAcsEntryThdRwRtStCshnFldUpwdDnwdPos_Val/1 -> Terminator_18/1
  PA_KeSMSw6sAcsEntryThdRwRtStFrwdBkwdPosMax_Val/1 -> Terminator_19/1
  PA_KeSMSw6sAcsEntryThdRwRtStFrwdBkwdPosMin_Val/1 -> Terminator_20/1
  PA_KeSMSw6sAcsEntryThdRwRtStFrwdBkwdPos_Val/1 -> Terminator_21/1
  PA_KeSMSw6sFamilyMdThdRwRtStFrwdBkwdPosMax_Val/1 -> Terminator_22/1
  PA_KeSMSw6sFamilyMdThdRwRtStFrwdBkwdPosMin_Val/1 -> Terminator_23/1
  PA_KeSMSw6sFamilyMdThdRwRtStFrwdBkwdPos_Val/1 -> Terminator_24/1
  PA_KeSMSw6sFamilyRMdThdRwRtStFrwdBkwdPosMax_Val/1 -> Terminator_25/1
  PA_KeSMSw6sFamilyRMdThdRwRtStFrwdBkwdPosMin_Val/1 -> Terminator_26/1
  PA_KeSMSw6sFamilyRMdThdRwRtStFrwdBkwdPos_Val/1 -> Terminator_27/1
  PA_KeSMSw6sLugThdRwRtStBkReclnUpwdDnwdPosMax_Val/1 -> Terminator_28/1
  PA_KeSMSw6sLugThdRwRtStBkReclnUpwdDnwdPosMin_Val/1 -> Terminator_29/1
  PA_KeSMSw6sLugThdRwRtStBkReclnUpwdDnwdPos_Val/1 -> Terminator_30/1
  PA_KeSMSw6sLugThdRwRtStCshnFldUpwdDnwdPosMax_Val/1 -> Terminator_31/1
  PA_KeSMSw6sLugThdRwRtStCshnFldUpwdDnwdPosMin_Val/1 -> Terminator_32/1
  PA_KeSMSw6sLugThdRwRtStCshnFldUpwdDnwdPos_Val/1 -> Terminator_33/1
  PA_KeSMSw6sLugThdRwRtStFrwdBkwdPosMax_Val/1 -> Terminator_34/1
  PA_KeSMSw6sLugThdRwRtStFrwdBkwdPosMin_Val/1 -> Terminator_35/1
  PA_KeSMSw6sLugThdRwRtStFrwdBkwdPos_Val/1 -> Terminator_36/1
  PA_KeSMSw6sVIPThdRwRtStBkReclnUpwdDnwdPosMax_Val/1 -> Terminator_37/1
  PA_KeSMSw6sVIPThdRwRtStBkReclnUpwdDnwdPosMin_Val/1 -> Terminator_38/1
  PA_KeSMSw6sVIPThdRwRtStBkReclnUpwdDnwdPos_Val/1 -> Terminator_39/1
  PA_KeSMSw6sVIPThdRwRtStFrwdBkwdPosMax_Val/1 -> Terminator_40/1
  PA_KeSMSw6sVIPThdRwRtStFrwdBkwdPosMin_Val/1 -> Terminator_41/1
  PA_KeSMSw6sVIPThdRwRtStFrwdBkwdPos_Val/1 -> Terminator_42/1
  PA_KeSMSwAcsEntryThdRwRtStBkReclnUpwdDnwdPosMax_Val/1 -> Terminator_43/1
  PA_KeSMSwAcsEntryThdRwRtStBkReclnUpwdDnwdPosMin_Val/1 -> Terminator_44/1
  PA_KeSMSwAcsEntryThdRwRtStBkReclnUpwdDnwdPos_Val/1 -> Terminator_45/1
  PA_KeSMSwAcsEntryThdRwRtStCshnFldUpwdDnwdPosMax_Val/1 -> Terminator_46/1
  PA_KeSMSwAcsEntryThdRwRtStCshnFldUpwdDnwdPosMin_Val/1 -> Terminator_47/1
  PA_KeSMSwAcsEntryThdRwRtStCshnFldUpwdDnwdPos_Val/1 -> Terminator_48/1
  PA_KeSMSwAcsEntryThdRwRtStFrwdBkwdPosMax_Val/1 -> Terminator_49/1
  PA_KeSMSwAcsEntryThdRwRtStFrwdBkwdPosMin_Val/1 -> Terminator_50/1
  PA_KeSMSwAcsEntryThdRwRtStFrwdBkwdPos_Val/1 -> Terminator_51/1
  PA_KeSMSwAcsMd53ThdRwRtBkReclnUpwdDnwdPosMax_Val/1 -> Terminator_52/1
  PA_KeSMSwAcsMd53ThdRwRtBkReclnUpwdDnwdPosMin_Val/1 -> Terminator_53/1
  PA_KeSMSwAcsMd53ThdRwRtBkReclnUpwdDnwdPos_Val/1 -> Terminator_54/1
  PA_KeSMSwAcsMd53ThdRwRtFldUpwdDnwdPosMax_Val/1 -> Terminator_55/1
  PA_KeSMSwAcsMd53ThdRwRtFldUpwdDnwdPosMin_Val/1 -> Terminator_56/1
  PA_KeSMSwAcsMd53ThdRwRtFldUpwdDnwdPos_Val/1 -> Terminator_57/1
  PA_KeSMSwAcsMd56ThdRwRtStBkReclnUpwdDnwdPosMax_Val/1 -> Terminator_58/1
  PA_KeSMSwAcsMd56ThdRwRtStBkReclnUpwdDnwdPosMin_Val/1 -> Terminator_59/1
  PA_KeSMSwAcsMd56ThdRwRtStBkReclnUpwdDnwdPos_Val/1 -> Terminator_60/1
  PA_KeSMSwAcsMd56ThdRwRtStCshnFldUpwdDnwdPosMax_Val/1 -> Terminator_61/1
  PA_KeSMSwAcsMd56ThdRwRtStCshnFldUpwdDnwdPosMin_Val/1 -> Terminator_62/1
  PA_KeSMSwAcsMd56ThdRwRtStCshnFldUpwdDnwdPos_Val/1 -> Terminator_63/1
  PA_KeSMSwAcsMd56ThdRwRtStFrwdBkwdPosMax_Val/1 -> Terminator_64/1
  PA_KeSMSwAcsMd56ThdRwRtStFrwdBkwdPosMin_Val/1 -> Terminator_65/1
  PA_KeSMSwAcsMd56ThdRwRtStFrwdBkwdPos_Val/1 -> Terminator_66/1
  PA_KeSMSwAcsMd57ThdRwRtStBkReclnUpwdDnwdPosMax_Val/1 -> Terminator_67/1
  PA_KeSMSwAcsMd57ThdRwRtStBkReclnUpwdDnwdPosMin_Val/1 -> Terminator_68/1
  PA_KeSMSwAcsMd57ThdRwRtStBkReclnUpwdDnwdPos_Val/1 -> Terminator_69/1
  PA_KeSMSwAcsMd57ThdRwRtStFrwdBkwdPosMax_Val/1 -> Terminator_70/1
  PA_KeSMSwAcsMd57ThdRwRtStFrwdBkwdPosMin_Val/1 -> Terminator_71/1
  PA_KeSMSwAcsMd57ThdRwRtStFrwdBkwdPos_Val/1 -> Terminator_72/1
  PA_KeSMSwAcsMd7ThdRwRtStBkReclnUpwdDnwdPosMax_Val/1 -> Terminator_73/1
  PA_KeSMSwAcsMd7ThdRwRtStBkReclnUpwdDnwdPosMin_Val/1 -> Terminator_74/1
  PA_KeSMSwAcsMd7ThdRwRtStBkReclnUpwdDnwdPos_Val/1 -> Terminator_75/1
  PA_KeSMSwAcsMd7ThdRwRtStCshnFldUpwdDnwdPosMax_Val/1 -> Terminator_76/1
  PA_KeSMSwAcsMd7ThdRwRtStCshnFldUpwdDnwdPosMin_Val/1 -> Terminator_77/1
  PA_KeSMSwAcsMd7ThdRwRtStCshnFldUpwdDnwdPos_Val/1 -> Terminator_78/1
  PA_KeSMSwAcsMd7ThdRwRtStFrwdBkwdPosMax_Val/1 -> Terminator_79/1
  PA_KeSMSwAcsMd7ThdRwRtStFrwdBkwdPosMin_Val/1 -> Terminator_80/1
  PA_KeSMSwAcsMd7ThdRwRtStFrwdBkwdPos_Val/1 -> Terminator_81/1
  PA_KeSMSwFamilyMdThdRwRtStFrwdBkwdPosMax_Val/1 -> Terminator_82/1
  PA_KeSMSwFamilyMdThdRwRtStFrwdBkwdPosMin_Val/1 -> Terminator_83/1
  PA_KeSMSwFamilyMdThdRwRtStFrwdBkwdPos_Val/1 -> Terminator_84/1
  PA_KeSMSwFamilyRMdThdRwRtStFrwdBkwdPosMax_Val/1 -> Terminator_85/1
  PA_KeSMSwFamilyRMdThdRwRtStFrwdBkwdPosMin_Val/1 -> Terminator_86/1
  PA_KeSMSwFamilyRMdThdRwRtStFrwdBkwdPos_Val/1 -> Terminator_87/1
  PA_KeSMSwLugThdRwRtStBkReclnUpwdDnwdPosMax_Val/1 -> Terminator_88/1
  PA_KeSMSwLugThdRwRtStBkReclnUpwdDnwdPosMin_Val/1 -> Terminator_89/1
  PA_KeSMSwLugThdRwRtStBkReclnUpwdDnwdPos_Val/1 -> Terminator_90/1
  PA_KeSMSwLugThdRwRtStCshnFldUpwdDnwdPosMax_Val/1 -> Terminator_91/1
  PA_KeSMSwLugThdRwRtStCshnFldUpwdDnwdPosMin_Val/1 -> Terminator_92/1
  PA_KeSMSwLugThdRwRtStCshnFldUpwdDnwdPos_Val/1 -> Terminator_93/1
  PA_KeSMSwLugThdRwRtStFrwdBkwdPosMax_Val/1 -> Terminator_94/1
  PA_KeSMSwLugThdRwRtStFrwdBkwdPosMin_Val/1 -> Terminator_95/1
  PA_KeSMSwLugThdRwRtStFrwdBkwdPos_Val/1 -> Terminator_96/1
  PA_KeSMSwVIPThdRwRtStBkReclnUpwdDnwdPosMax_Val/1 -> Terminator_97/1
  PA_KeSMSwVIPThdRwRtStBkReclnUpwdDnwdPosMin_Val/1 -> Terminator_98/1
  PA_KeSMSwVIPThdRwRtStBkReclnUpwdDnwdPos_Val/1 -> Terminator_99/1
  PA_KeSMSwVIPThdRwRtStFrwdBkwdPosMax_Val/1 -> Terminator_100/1
  PA_KeSMSwVIPThdRwRtStFrwdBkwdPosMin_Val/1 -> Terminator_101/1
  PA_KeSMSwVIPThdRwRtStFrwdBkwdPos_Val/1 -> Terminator_102/1

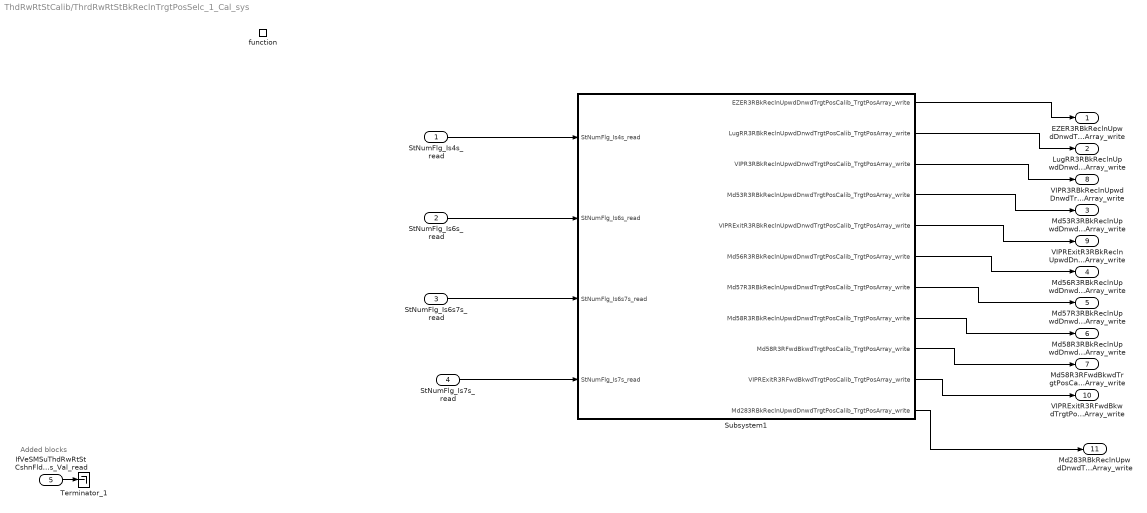
== system ThdRwRtStCalib/ThrdRwRtStBkReclnTrgtPosSelc_1_Cal_sys ==
  note: Added blocks
  StNumFlg_Is4s_read : Inport
  StNumFlg_Is6s_read : Inport  Port=2
  StNumFlg_Is6s7s_read : Inport  Port=3
  StNumFlg_Is7s_read : Inport  Port=4
  IfVeSMSuThdRwRtStCshnFldUpwdDnwdPos_Val_read : Inport  Port=5
  function : TriggerPort  TriggerType=function-call  IsSimulinkFunction=on  FunctionName=ThrdRwRtStBkReclnTrgtPosSelc_1_Cal  VariantControl=(inherit)
  Subsystem1 : Subsystem
  Terminator_1 : Terminator
  EZER3RBkReclnUpwdDnwdTrgtPosCalib_TrgtPosArray_write : Outport  VectorParamsAs1DForOutWhenUnconnected=off
  LugRR3RBkReclnUpwdDnwdTrgtPosCalib_TrgtPosArray_write : Outport  Port=2  VectorParamsAs1DForOutWhenUnconnected=off
  Md53R3RBkReclnUpwdDnwdTrgtPosCalib_TrgtPosArray_write : Outport  Port=3  VectorParamsAs1DForOutWhenUnconnected=off
  Md56R3RBkReclnUpwdDnwdTrgtPosCalib_TrgtPosArray_write : Outport  Port=4  VectorParamsAs1DForOutWhenUnconnected=off
  Md57R3RBkReclnUpwdDnwdTrgtPosCalib_TrgtPosArray_write : Outport  Port=5  VectorParamsAs1DForOutWhenUnconnected=off
  Md58R3RBkReclnUpwdDnwdTrgtPosCalib_TrgtPosArray_write : Outport  Port=6  VectorParamsAs1DForOutWhenUnconnected=off
  Md58R3RFwdBkwdTrgtPosCalib_TrgtPosArray_write : Outport  Port=7  VectorParamsAs1DForOutWhenUnconnected=off
  VIPR3RBkReclnUpwdDnwdTrgtPosCalib_TrgtPosArray_write : Outport  Port=8  VectorParamsAs1DForOutWhenUnconnected=off
  VIPRExitR3RBkReclnUpwdDnwdTrgtPosCalib_TrgtPosArray_write : Outport  Port=9  VectorParamsAs1DForOutWhenUnconnected=off
  VIPRExitR3RFwdBkwdTrgtPosCalib_TrgtPosArray_write : Outport  Port=10  VectorParamsAs1DForOutWhenUnconnected=off
  Md283RBkReclnUpwdDnwdTrgtPosCalib_TrgtPosArray_write : Outport  Port=11  VectorParamsAs1DForOutWhenUnconnected=off
      settings: EnsureOutportIsVirtual=on
  wires:
  StNumFlg_Is4s_read/1 -> Subsystem1/1(StNumFlg_Is4s_read)
  StNumFlg_Is6s_read/1 -> Subsystem1/2(StNumFlg_Is6s_read)
  StNumFlg_Is6s7s_read/1 -> Subsystem1/3(StNumFlg_Is6s7s_read)
  Subsystem1/1(EZER3RBkReclnUpwdDnwdTrgtPosCalib_TrgtPosArray_write) -> EZER3RBkReclnUpwdDnwdTrgtPosCalib_TrgtPosArray_write/1
  Subsystem1/2(LugRR3RBkReclnUpwdDnwdTrgtPosCalib_TrgtPosArray_write) -> LugRR3RBkReclnUpwdDnwdTrgtPosCalib_TrgtPosArray_write/1
  Subsystem1/3(VIPR3RBkReclnUpwdDnwdTrgtPosCalib_TrgtPosArray_write) -> VIPR3RBkReclnUpwdDnwdTrgtPosCalib_TrgtPosArray_write/1
  Subsystem1/4(Md53R3RBkReclnUpwdDnwdTrgtPosCalib_TrgtPosArray_write) -> Md53R3RBkReclnUpwdDnwdTrgtPosCalib_TrgtPosArray_write/1
  Subsystem1/5(VIPRExitR3RBkReclnUpwdDnwdTrgtPosCalib_TrgtPosArray_write) -> VIPRExitR3RBkReclnUpwdDnwdTrgtPosCalib_TrgtPosArray_write/1
  Subsystem1/6(Md56R3RBkReclnUpwdDnwdTrgtPosCalib_TrgtPosArray_write) -> Md56R3RBkReclnUpwdDnwdTrgtPosCalib_TrgtPosArray_write/1
  Subsystem1/7(Md57R3RBkReclnUpwdDnwdTrgtPosCalib_TrgtPosArray_write) -> Md57R3RBkReclnUpwdDnwdTrgtPosCalib_TrgtPosArray_write/1
  Subsystem1/8(Md58R3RBkReclnUpwdDnwdTrgtPosCalib_TrgtPosArray_write) -> Md58R3RBkReclnUpwdDnwdTrgtPosCalib_TrgtPosArray_write/1
  Subsystem1/9(Md58R3RFwdBkwdTrgtPosCalib_TrgtPosArray_write) -> Md58R3RFwdBkwdTrgtPosCalib_TrgtPosArray_write/1
  Subsystem1/10(VIPRExitR3RFwdBkwdTrgtPosCalib_TrgtPosArray_write) -> VIPRExitR3RFwdBkwdTrgtPosCalib_TrgtPosArray_write/1
  Subsystem1/11(Md283RBkReclnUpwdDnwdTrgtPosCalib_TrgtPosArray_write) -> Md283RBkReclnUpwdDnwdTrgtPosCalib_TrgtPosArray_write/1
  StNumFlg_Is7s_read/1 -> Subsystem1/4(StNumFlg_Is7s_read)
  IfVeSMSuThdRwRtStCshnFldUpwdDnwdPos_Val_read/1 -> Terminator_1/1

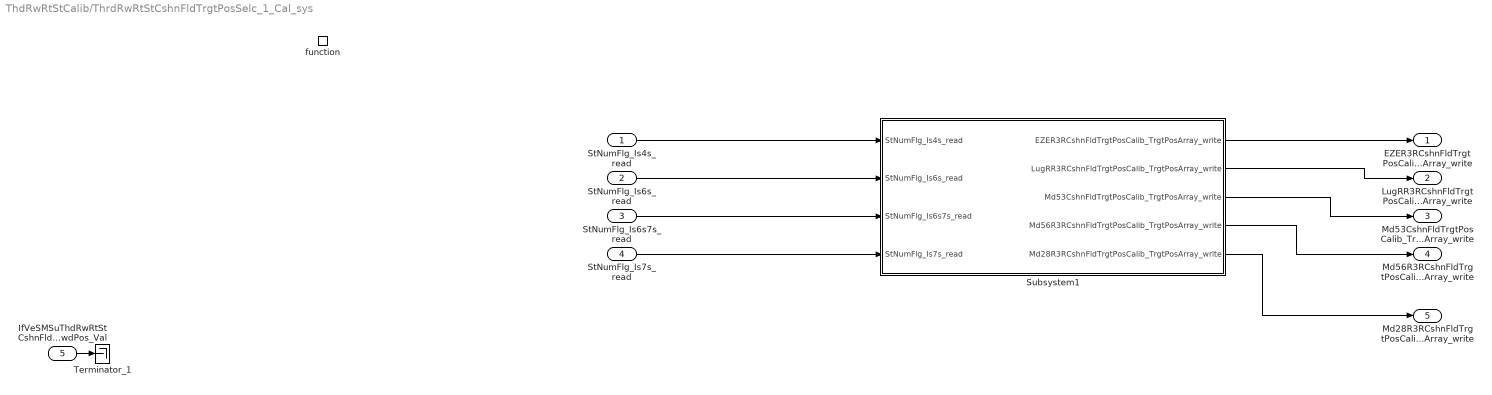
== system ThdRwRtStCalib/ThrdRwRtStCshnFldTrgtPosSelc_1_Cal_sys ==
  StNumFlg_Is4s_read : Inport
  StNumFlg_Is6s_read : Inport  Port=2
  StNumFlg_Is6s7s_read : Inport  Port=3
  StNumFlg_Is7s_read : Inport  Port=4
  IfVeSMSuThdRwRtStCshnFldUpwdDnwdPos_Val : Inport  Port=5
  function : TriggerPort  TriggerType=function-call  IsSimulinkFunction=on  FunctionName=ThrdRwRtStCshnFldTrgtPosSelc_1_Cal  VariantControl=(inherit)
  Subsystem1 : Subsystem
  Terminator_1 : Terminator
  EZER3RCshnFldTrgtPosCalib_TrgtPosArray_write : Outport  VectorParamsAs1DForOutWhenUnconnected=off
  LugRR3RCshnFldTrgtPosCalib_TrgtPosArray_write : Outport  Port=2  VectorParamsAs1DForOutWhenUnconnected=off
  Md53CshnFldTrgtPosCalib_TrgtPosArray_write : Outport  Port=3  VectorParamsAs1DForOutWhenUnconnected=off
  Md56R3RCshnFldTrgtPosCalib_TrgtPosArray_write : Outport  Port=4  VectorParamsAs1DForOutWhenUnconnected=off
  Md28R3RCshnFldTrgtPosCalib_TrgtPosArray_write : Outport  Port=5  VectorParamsAs1DForOutWhenUnconnected=off
      settings: EnsureOutportIsVirtual=on
  wires:
  Subsystem1/1(EZER3RCshnFldTrgtPosCalib_TrgtPosArray_write) -> EZER3RCshnFldTrgtPosCalib_TrgtPosArray_write/1
  Subsystem1/2(LugRR3RCshnFldTrgtPosCalib_TrgtPosArray_write) -> LugRR3RCshnFldTrgtPosCalib_TrgtPosArray_write/1
  Subsystem1/3(Md53CshnFldTrgtPosCalib_TrgtPosArray_write) -> Md53CshnFldTrgtPosCalib_TrgtPosArray_write/1
  Subsystem1/4(Md56R3RCshnFldTrgtPosCalib_TrgtPosArray_write) -> Md56R3RCshnFldTrgtPosCalib_TrgtPosArray_write/1
  StNumFlg_Is4s_read/1 -> Subsystem1/1(StNumFlg_Is4s_read)
  StNumFlg_Is6s_read/1 -> Subsystem1/2(StNumFlg_Is6s_read)
  StNumFlg_Is6s7s_read/1 -> Subsystem1/3(StNumFlg_Is6s7s_read)
  StNumFlg_Is7s_read/1 -> Subsystem1/4(StNumFlg_Is7s_read)
  Subsystem1/5(Md28R3RCshnFldTrgtPosCalib_TrgtPosArray_write) -> Md28R3RCshnFldTrgtPosCalib_TrgtPosArray_write/1
  IfVeSMSuThdRwRtStCshnFldUpwdDnwdPos_Val/1 -> Terminator_1/1
